simulink model "TimingTest"  (R2024b)
settings: Solver=VariableStepAuto  StartTime=0.0  StopTime=.01  RelTol=1e-3
libraries: simulink x2
settings Model: Creator=oxbro  LastModifiedBy=oxbro

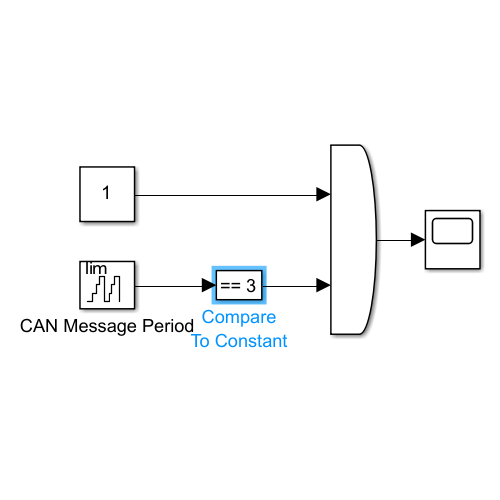
[thumbnail: Simulink's stored preview of the top-level diagram]
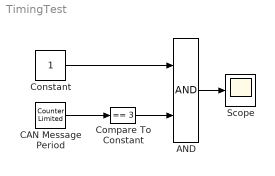
== system TimingTest ==
  AND : Logic  IconShape=distinctive  AllPortsSameDT=off  OutDataTypeStr=boolean
  CAN Message Period : simulink/Sources/Counter Limited  uplimit=4  tsamp=.001
  Compare To Constant : simulink/Logic and Bit Operations/Compare To Constant  relop===  const=3  OutDataTypeStr=boolean
  Constant : Constant
  Scope : Scope
  wires:
  AND/1 -> Scope/1
  Compare To Constant/1 -> AND/2
  CAN Message Period/1 -> Compare To Constant/1
  Constant/1 -> AND/1
